simulink model "white_noise_spectrum"  (R2024a)
settings: Solver=VariableStepAuto  StartTime=0.0  StopTime=50.0  RelTol=1e-3
libraries: simulink x4, simulink_extras x4
settings Model: Creator=evgenijkondratev  LastModifiedBy=evgenijkondratev

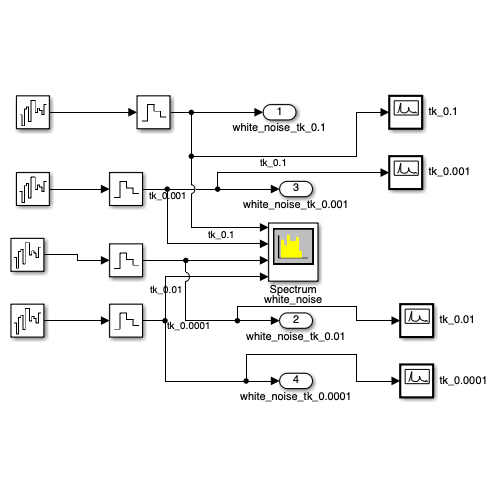
[thumbnail: Simulink's stored preview of the top-level diagram]
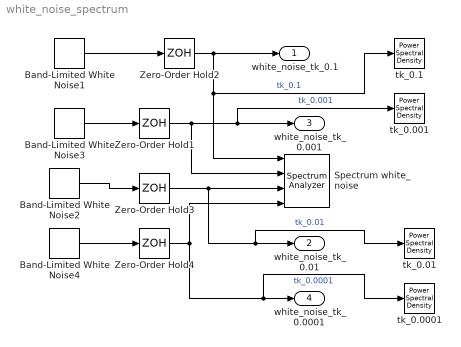
== system white_noise_spectrum ==
  Band-Limited White Noise1 : simulink/Sources/Band-Limited White Noise  Cov=[1]  Ts=0.1  seed=[23341]
  Band-Limited White Noise2 : simulink/Sources/Band-Limited White Noise  Cov=[1]  Ts=0.01  seed=[23341]
  Band-Limited White Noise3 : simulink/Sources/Band-Limited White Noise  Cov=[1]  Ts=0.001  seed=[23341]
  Band-Limited White Noise4 : simulink/Sources/Band-Limited White Noise  Cov=[1]  Ts=0.0001  seed=[23341]
  Spectrum white_noise : SpectrumAnalyzer  NumInputPorts=4  WindowPosition=[170.000000,173.000000,1565.000000,787.000000,]  ScopeFrameLocation=window  YLimits=[-45.50570639,51.96680639]  ShowLegend=on
  Zero-Order Hold{1..4} (4 alike) : ZeroOrderHold  SampleTime=0.001
  tk_0.0001 : simulink_extras/Additional Sinks/Power Spectral Density  npts=128  fftpts=512  HowOften=64  sampleT=0.1
  tk_0.001 : simulink_extras/Additional Sinks/Power Spectral Density  npts=128  fftpts=512  HowOften=64  sampleT=0.1
  tk_0.01 : simulink_extras/Additional Sinks/Power Spectral Density  npts=128  fftpts=512  HowOften=64  sampleT=0.1
  tk_0.1 : simulink_extras/Additional Sinks/Power Spectral Density  npts=128  fftpts=512  HowOften=64  sampleT=0.1
  white_noise_tk_0.1 : Outport
  white_noise_tk_0.01 : Outport  Port=2
  white_noise_tk_0.001 : Outport  Port=3
  white_noise_tk_0.0001 : Outport  Port=4
  wires:
  Zero-Order Hold3/1 -> tk_0.01/1, white_noise_tk_0.01/1, Spectrum white_noise/3  "tk_0.01"
  Zero-Order Hold2/1 -> tk_0.1/1, Spectrum white_noise/1, white_noise_tk_0.1/1  "tk_0.1"
  Band-Limited White Noise2/1 -> Zero-Order Hold3/1
  Band-Limited White Noise1/1 -> Zero-Order Hold2/1
  Band-Limited White Noise3/1 -> Zero-Order Hold1/1
  Zero-Order Hold1/1 -> tk_0.001/1, white_noise_tk_0.001/1, Spectrum white_noise/2  "tk_0.001"
  Band-Limited White Noise4/1 -> Zero-Order Hold4/1
  Zero-Order Hold4/1 -> tk_0.0001/1, white_noise_tk_0.0001/1, Spectrum white_noise/4  "tk_0.0001"
